simulink model "modelo3"  (Simulink 7.5)
settings: Solver=ode45  StartTime=0.0  StopTime=10  RelTol=1e-3
values from neighbouring files (symbols this model uses):
  Hz = 10    [modelo_controlador_analisis.m]
  rr = 1    [modelo_controlador_analisis.m]
  T = 0.02    [modelo_controlador_analisis.m]
libraries: simulink x1
settings Model: Creator=n421  LastModifiedBy=n421  CovModelRefEnable=off
settings DataIOCC: SaveFormat=StructureWithTime
settings OptimizationCC: ExpressionDepthLimit=128
settings DebuggingCC: UnderspecifiedInitializationDetection=Simplified  MergeDetectMultiDrivingBlocksExec=error  SolverPrmCheckMsg=none  FcnCallInpInsideContextMsg=Enable All  StateNameClashWarn=none
settings HardwareCC: ProdIntDivRoundTo=Zero  ProdEndianess=LittleEndian  ProdHWDeviceType=Specified
settings CodeAppCC: CustomSymbolStrType=$N$R$M_T
settings GRTTargetCC: TargetFunctionLibrary=C89/C90 (ANSI)  GeneratePreprocessorConditionals=Use local settings

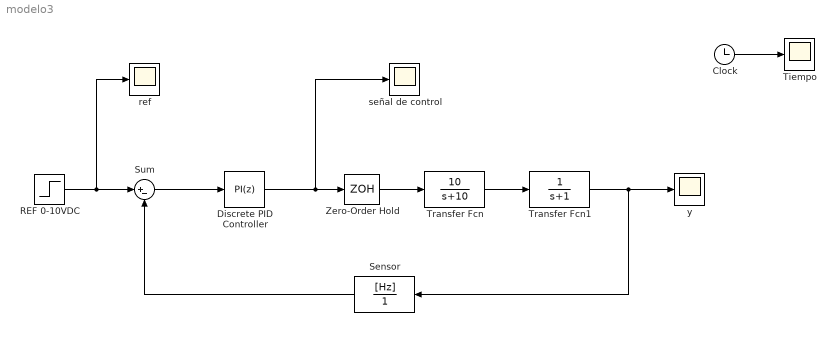
== system modelo3 ==
  Clock : Clock
  Discrete PID Controller : simulink/Continuous/PID Controller  Controller=PI  TimeDomain=Discrete-time  SampleTime=T  IntegratorMethod=Trapezoidal  FilterMethod=Forward Euler  Form=Parallel  UseFilter=on  ControllerParametersSource=internal  P=0.8511  I=0.5881  D=0  N=100  InitialConditionSource=internal  InitialConditionForIntegrator=0  InitialConditionForFilter=0  ExternalReset=none  LimitOutput=off  UpperSaturationLimit=inf  LowerSaturationLimit=-inf  LinearizeAsGain=off  AntiWindupMode=none  Kb=1  TrackingMode=off  Kt=1  PParamMin=[]  PParamMax=[]  IParamMin=[]  IParamMax=[]  DParamMin=[]  DParamMax=[]  NParamMin=[]  NParamMax=[]  KbParamMin=[]  KbParamMax=[]  KtParamMin=[]  KtParamMax=[]  POutMin=[]  POutMax=[]  IOutMin=[]  IOutMax=[]  DOutMin=[]  DOutMax=[]  NOutMin=[]  NOutMax=[]  KbOutMin=[]  KbOutMax=[]  KtOutMin=[]  KtOutMax=[]  IntegratorOutMin=[]  IntegratorOutMax=[]  FilterOutMin=[]  FilterOutMax=[]  SumOutMin=[]  SumOutMax=[]  SumI1OutMin=[]  SumI1OutMax=[]  SumI2OutMin=[]  SumI2OutMax=[]  SumI3OutMin=[]  SumI3OutMax=[]  SumDOutMin=[]  SumDOutMax=[]  SaturationOutMin=[]  SaturationOutMax=[]  IntegratorContinuousStateAttributes=''  IntegratorStateMustResolveToSignalObject=off  IntegratorRTWStateStorageClass=Auto  FilterContinuousStateAttributes=''  FilterStateMustResolveToSignalObject=off  FilterRTWStateStorageClass=Auto  DifferentiatorICPrevScaledInput=0  DifferentiatorOutMin=[]  DifferentiatorOutMax=[]
  REF 0-10VDC : Step  Time=0  After=rr  SampleTime=0
  Sensor : DiscreteTransferFcn  Numerator=[Hz]  Denominator=[1]  SampleTime=T
  Sum : Sum  Inputs=|+-
  "Tiempo " : Scope
      settings: TimeRange=auto  MaxDataPoints=5000  SaveName=tiempo  YMin=-1.25  YMax=11.25  SampleTime=-1  DataFormat=Array
  Transfer Fcn : TransferFcn  Numerator=[10]  Denominator=[1 10]
  Transfer Fcn1 : TransferFcn  Denominator=[1 1]
  Zero-Order Hold : ZeroOrderHold  SampleTime=T
  ref : Scope
      settings: TimeRange=auto  MaxDataPoints=5000  SaveName=r  YMin=0.9  YMax=1.1  SampleTime=-1  DataFormat=Array
  señal de control : Scope
      settings: TimeRange=auto  MaxDataPoints=5000  SaveName=u  YMin=-0.13264  YMax=0.96694  SampleTime=-1  DataFormat=Array
  y : Scope
      settings: TimeRange=auto  MaxDataPoints=5000  SaveName=y  YMin=-0.01406  YMax=0.12652  SampleTime=-1  DataFormat=Array
  wires:
  Transfer Fcn1/1 -> Sensor/1, y/1
  Sum/1 -> Discrete PID Controller/1
  Zero-Order Hold/1 -> Transfer Fcn/1
  Transfer Fcn/1 -> Transfer Fcn1/1
  Sensor/1 -> Sum/2
  REF 0-10VDC/1 -> ref/1, Sum/1
  Discrete PID Controller/1 -> señal de control/1, Zero-Order Hold/1
  Clock/1 -> "Tiempo "/1
